simulink model "DC_MOTOR"  (R2018a)
settings: Solver=VariableStepAuto  StartTime=0.0  StopTime=35  RelTol=1e-3
model workspace (MAT data in the model file):
  B = 2.69254913662e-19
  J = 0.000262842480729
  K = 0.01323780842
  L = 0.00192532731313
  R = 0.08
libraries: simulink x3, simulink_extras x2
settings Model: Creator=Hazem Elwakeel  LastModifiedBy=Hazem Elwakeel

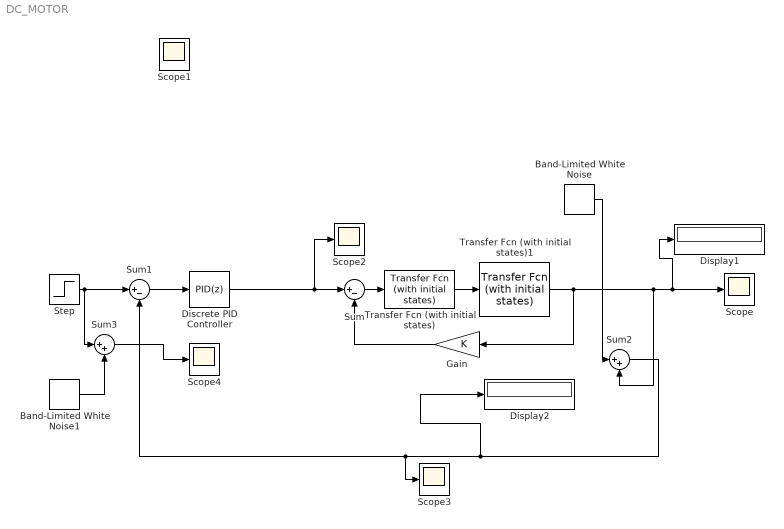
== system DC_MOTOR ==
  Band-Limited White Noise : simulink/Sources/Band-Limited White Noise  Cov=[0]  Ts=0.1  seed=[23341]
  Band-Limited White Noise1 : simulink/Sources/Band-Limited White Noise  Cov=[10]  Ts=0.1  seed=[23341]
  Discrete PID Controller : simulink/Continuous/PID Controller  Controller=PID  TimeDomain=Discrete-time  SampleTime=0.1  IntegratorMethod=Forward Euler  FilterMethod=Forward Euler  Form=Parallel  UseFilter=on  ControllerParametersSource=internal  P=0.00151160857606304  I=0.0302321715212607  D=0  N=100  InitialConditionSource=internal  InitialConditionForIntegrator=0  InitialConditionForFilter=0  ExternalReset=none  LimitOutput=on  UpperSaturationLimit=13  LowerSaturationLimit=0  LinearizeAsGain=off  AntiWindupMode=back-calculation  Kb=1  TrackingMode=off  Kt=1  PParamMin=[]  PParamMax=[]  IParamMin=[]  IParamMax=[]  DParamMin=[]  DParamMax=[]  NParamMin=[]  NParamMax=[]  KbParamMin=[]  KbParamMax=[]  KtParamMin=[]  KtParamMax=[]  POutMin=[]  POutMax=[]  IOutMin=[]  IOutMax=[]  DOutMin=[]  DOutMax=[]  NOutMin=[]  NOutMax=[]  KbOutMin=[]  KbOutMax=[]  KtOutMin=[]  KtOutMax=[]  IntegratorOutMin=[]  IntegratorOutMax=[]  FilterOutMin=[]  FilterOutMax=[]  SumOutMin=[]  SumOutMax=[]  SumI1OutMin=[]  SumI1OutMax=[]  SumI2OutMin=[]  SumI2OutMax=[]  SumI3OutMin=[]  SumI3OutMax=[]  SumDOutMin=[]  SumDOutMax=[]  SaturationOutMin=[]  SaturationOutMax=[]  IntegratorContinuousStateAttributes=''  IntegratorStateMustResolveToSignalObject=off  IntegratorRTWStateStorageClass=Auto  FilterContinuousStateAttributes=''  FilterStateMustResolveToSignalObject=off  FilterRTWStateStorageClass=Auto  DifferentiatorICPrevScaledInput=0  DifferentiatorOutMin=[]  DifferentiatorOutMax=[]  FilterDiffOutCoefMin=[]  FilterDiffOutCoefMax=[]  SumDenOutMin=[]  SumDenOutMax=[]  SumNumOutMin=[]  SumNumOutMax=[]  ReciprocalOutMin=[]  ReciprocalOutMax=[]  DivideOutMin=[]  DivideOutMax=[]  TunerSelectOption=Transfer Function Based (PID Tuner App)
  Display1 : Display
  Display2 : Display
  Gain : Gain  Gain=K
  Scope{,1..4} (5 alike) : Scope
  Step : Step  Time=0  After=500  SampleTime=0
  Sum : Sum  Inputs=|+-
  Sum1 : Sum  Inputs=|+-
  Sum2 : Sum  Inputs=|++
  Sum3 : Sum  Inputs=|++
  Transfer Fcn (with initial states) : simulink_extras/Additional Linear/Transfer Fcn (with initial states)  N=[K]  D="[J  B]"  X0=.5
  Transfer Fcn (with initial states)1 : simulink_extras/Additional Linear/Transfer Fcn (with initial states)  N=[1]  D="[L  R]"  X0=.5
  wires:
  Transfer Fcn (with initial states)/1 -> Transfer Fcn (with initial states)1/1
  Sum/1 -> Transfer Fcn (with initial states)/1
  Gain/1 -> Sum/2
  Transfer Fcn (with initial states)1/1 -> Gain/1, Display1/1, Scope/1, Sum2/2
  Sum1/1 -> Discrete PID Controller/1
  Step/1 -> Sum3/1, Sum1/1
  Discrete PID Controller/1 -> Scope2/1, Sum/1
  Sum2/1 -> Display2/1, Scope3/1, Sum1/2
  Band-Limited White Noise/1 -> Sum2/1
  Band-Limited White Noise1/1 -> Sum3/2
  Sum3/1 -> Scope4/1
